simulink model "example"  (Simulink 7.6)
settings: Solver=ode4  StartTime=0.0  StopTime=inf  FixedStep=0.01  RelTol=1e-3
libraries: LUCAS x1, aerolibanimutils x1
settings Model: Creator=ttcl3  LastModifiedBy=Owen

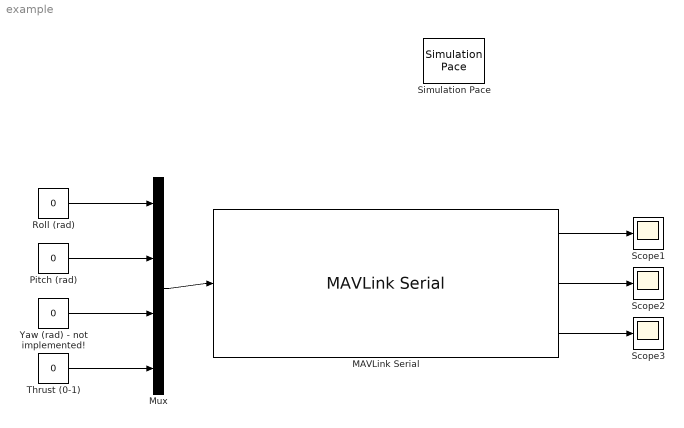
== system example ==
  MAVLink Serial : LUCAS/MAVLink Serial  COM_Port='COM5'  Baud_Rate=57600  HEART_BEAT=off  ATTITUDE_OUT=on  RAW_IMU=off  POSITION_OUT=on  VFR_HUD=on  RC_SCALED=off  SERVO_OUT_RAW=off  SET_MODE=off  DATA_STREAM=off  ATTITUDE_COMMAND=on  ATTITUDE_IN=off  GPS_RAW_IN=off  VFR_HUD_IN=off
  Mux : Mux
  Pitch (rad) : Constant  Value=0
  Roll (rad) : Constant  Value=0
  Scope1 : Scope
      settings: YMin=-0.1  YMax=0.1
  Scope2 : Scope
      settings: YMin=-0.85  YMax=0.15
  Scope3 : Scope
      settings: YMin=-0.85  YMax=0.15  SaveName=ScopeData3
  Simulation Pace : aerolibanimutils/Simulation Pace  SimulationPace=1  SleepMode=MATLAB Thread  OutputPaceError=off  SampleTime=0.01
      settings: AttributesFormatString=%<SimulationPace> sec/sec
  Thrust (0-1) : Constant  Value=0
  Yaw (rad) - not implemented! : Constant  Value=0
  wires:
  Mux/1 -> MAVLink Serial/1
  Roll (rad)/1 -> Mux/1
  Pitch (rad)/1 -> Mux/2
  Yaw (rad) - not implemented!/1 -> Mux/3
  Thrust (0-1)/1 -> Mux/4
  MAVLink Serial/1 -> Scope1/1
  MAVLink Serial/2 -> Scope2/1
  MAVLink Serial/3 -> Scope3/1
